simulink model "ekf2mlf"  (R2014a)
settings: Solver=FixedStepDiscrete  StartTime=0.0  StopTime=100.0  RelTol=1e-3
values from neighbouring files (symbols this model uses):
  T = block.DialogPrm(6).Data    [sfall2.m]    (also in sysall.m = 0.05)
undefined symbols (not defined in the file or in its folder): phi_0, psi_0, Q, R, theta_0, V_0
libraries: simulink x3
settings Model: Creator=gcampa  LastModifiedBy=gcampa
settings DataIOCC: SignalLoggingSaveFormat=ModelDataLogs  SaveOutput=off  SignalLogging=off  DSMLogging=off  SaveTime=off
settings OptimizationCC: ExpressionDepthLimit=2147483647  InitFltsAndDblsToZero=on
settings DebuggingCC: SaveWithParameterizedLinksMsg=none  UnderspecifiedInitializationDetection=Classic  SignalResolutionControl=TryResolveAllWithWarning  MultiTaskDSMMsg=warning  MultiTaskCondExecSysMsg=none  FcnCallInpInsideContextMsg=UseLocalSettings  StateNameClashWarn=warning
settings SFSimCC: SimParseCustomCode=off
settings RTWCC: IncludeERTFirstTime=on  RTWCompilerOptimization=On
settings GRTTargetCC: TargetFcnLib=ansi_tfl_tmw.mat  CombineOutputUpdateFcns=off  GRTInterface=on

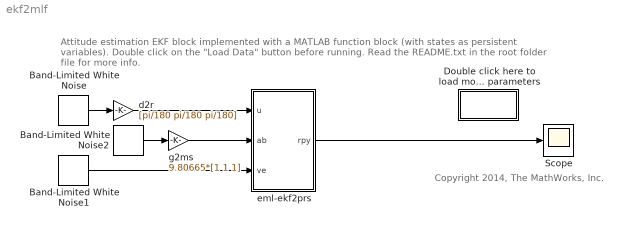
== system ekf2mlf ==
  note: Attitude estimation EKF block implemented with a MATLAB function block (with states as persistent variables).
      | Double click on the "Load Data" button before running. Read the README.txt in the root folder file for more info.
  note: Copyright 2014, The MathWorks, Inc.
  Band-Limited White Noise : simulink/Sources/Band-Limited White Noise  Cov=0.1*[1 1 1]  Ts=T  seed=[1 2 3]
  Band-Limited White Noise1 : simulink/Sources/Band-Limited White Noise  Cov=0.1*[1 1 1]  Ts=T  seed=[7 8 9]
  Band-Limited White Noise2 : simulink/Sources/Band-Limited White Noise  Cov=0.1*[1 1 1]  Ts=T  seed=[4 5 6]
  Double click here to load model and parameters : Subsystem
      settings: OpenFcn=|
      | V_0= 21.44176640107837;
      | phi_0=0.16673723163960;
      | theta_0=0.38249284705297;
      | psi_0=-3.10672050096899;
      | 
      | Q= [1.1339e-006     0               0
      |     0               3.1232e-006     0
      |     0               0               2.9009e-006];
      | 
      | R= [0.3368          0               0
      |     0               0.092           0
      |     0               0               0];
      | 
      | T=0.05;
      mask Display: disp('Load\nData')
  Scope : Scope
      settings: TimeRange=100  YMin=-4  YMax=4
  d2r : Gain  Gain=[pi/180 pi/180 pi/180]  SaturateOnIntegerOverflow=on  OutDataTypeStr=Inherit: Same as input  ParamDataTypeStr=Inherit: Same as input
  eml-ekf2prs : MATLAB Function  TreatAsAtomicUnit=on
  g2ms : Gain  Gain=9.80665*[1 1 1]  SaturateOnIntegerOverflow=on  OutDataTypeStr=Inherit: Same as input  ParamDataTypeStr=Inherit: Same as input
  wires:
  Band-Limited White Noise/1 -> d2r/1
  Band-Limited White Noise1/1 -> eml-ekf2prs/3(ve)
  Band-Limited White Noise2/1 -> g2ms/1
  eml-ekf2prs/1(rpy) -> Scope/1
  d2r/1 -> eml-ekf2prs/1(u)
  g2ms/1 -> eml-ekf2prs/2(ab)

== system ekf2mlf/Double click here to load model and parameters ==

== matlab function ekf2mlf/eml-ekf2prs ==
  data: u input; ab input; ve input; rpy output; Q parameter; R parameter; phi_0 parameter; theta_0 parameter; psi_0 parameter; T parameter; V_0 parameter
function rpy=ekf2prs(u,ab,ve,Q, R,phi_0,theta_0,psi_0,T,V_0)

%% initialization

% constants
W=Q(1:2,1:2);
V=R(1:2,1:2);
Plim=1e-5;

% state variables
persistent P x vold
if isempty(P) || isempty(x) || isempty(vold),
    P=zeros(2);
    x=[phi_0 theta_0]';
    vold=[V_0*cos(psi_0) V_0*sin(psi_0) V_0*sin(theta_0)]';
end

%% Calculate rpy as a function of inputs and state.

% calculate heading
psi=atan2(ve(2),ve(1));

% attach psi to x and send all to output
rpy = [x;psi];


%% Calculate next state

% calculate gps acceleration
agps = (ve-vold)/T;

% rotate gps acceleration
rx=-cos(psi)*agps(1)-sin(psi)*agps(2);
ry=sin(psi)*agps(1)-cos(psi)*agps(2);
rz=9.80665-agps(3);

% solve for theta and phi given imu and gps accelerations
sth=(rx*ab(1)+rz*(abs(rx^2+rz^2-ab(1)^2)^0.5))/(realmin+rx^2+rz^2);
theta=atan2(sth*rx-ab(1),sth*rz);
rth=rx*sin(theta)+rz*cos(theta);
sph=(ry*ab(2)+rth*(abs(ry^2+rth^2-ab(2)^2)^0.5))/(realmin+ry^2+rth^2);
phi=atan2(-sph*ry+ab(2),sph*rth);

% this works as the "measured" output in the ekf
y = [phi;theta];

% states (note, phi and theta are re-initialized with the previous estimates)
phi=x(1);
theta=x(2);

% inputs
p=u(1);
q=u(2);
r=u(3);

% omega to attitude dot
Taw=[1 sin(phi)*tan(theta) cos(phi)*tan(theta); 0 cos(phi) -sin(phi)];

% x propagation
xdot=Taw*[p;q;r];
xm=x+T*xdot;

% A matrix
a = [ cos(phi)*tan(theta)*q-sin(phi)*tan(theta)*r      sin(phi)*(1+tan(theta)^2)*q+cos(phi)*(1+tan(theta)^2)*r
      -sin(phi)*q-cos(phi)*r                           0                                                      ];

% euler forward step
A = eye(2)+T*a; 

% find K

Pm=W+A*P*A';
VPm=V+Pm;
VPm_det=VPm(1,1)*VPm(2,2)-VPm(1,2)*VPm(2,1);
iVPm=[VPm(2,2) -VPm(1,2); -VPm(2,1) VPm(1,1)]/VPm_det;
K=Pm*iVPm;

% EKF update equations
Pp=(eye(2)-K)*Pm;
xp=xm+K*(y-xm);

% ball norm limiter
nrm=sqrt(Pp(:)'*Pp(:));
Pp=Pp*min(nrm,Plim)/max(nrm,realmin);

% store
P = Pp;
x = xp;
vold = ve;
